simulink subsystem "Day1_Scenario_3_4"  (R2024a)
settings: Solver=VariableStepAuto  StartTime=0.0  StopTime=10.0  RelTol=1e-3
libraries: CarMaker4SL x3
settings Model: Creator=junhyung.cha  LastModifiedBy=User

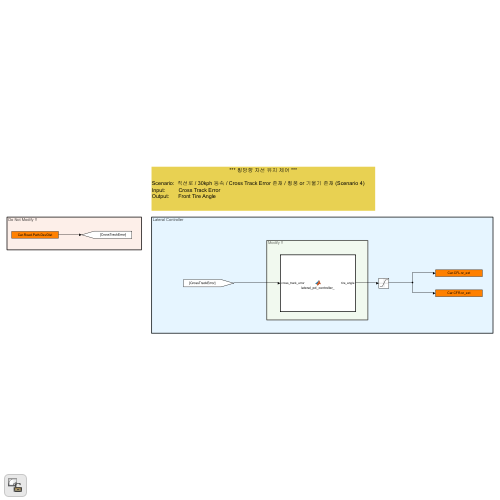
[thumbnail: Simulink's stored preview of the top-level diagram]
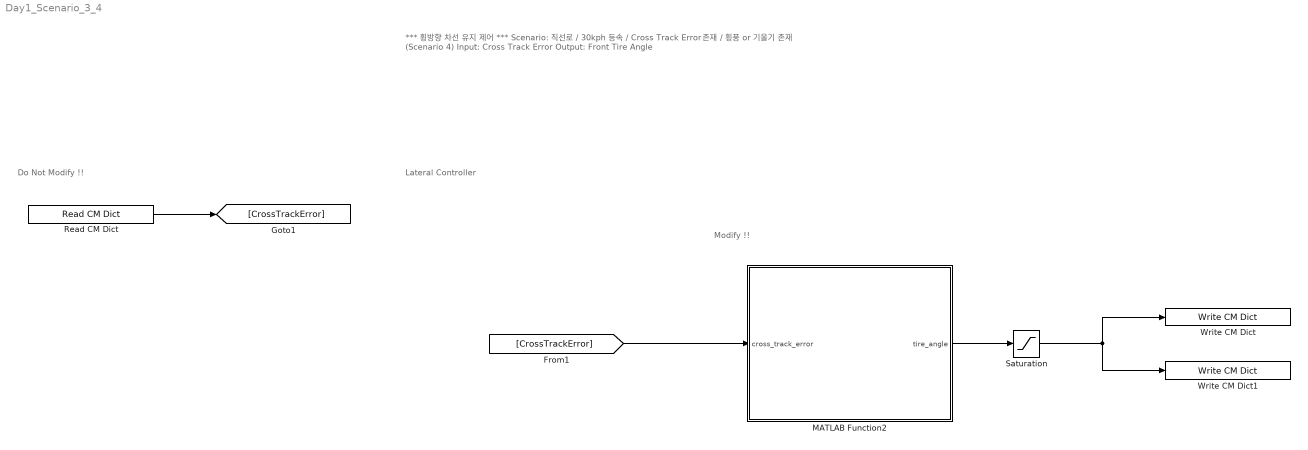
== system Day1_Scenario_3_4 ==
  note: Do Not Modify !!
  note: Modify !!
  note: Lateral Controller
  note: *** 횡방향 차선 유지 제어 ***
      |
      | Scenario: 직선로 / 30kph 등속 / Cross Track Error 존재 / 횡풍 or 기울기 존재 (Scenario 4)
      | Input: Cross Track Error
      | Output: Front Tire Angle
  MATLAB Function2 : MATLAB Function  TreatAsAtomicUnit=on
  Read CM Dict : CarMaker4SL/Read CM Dict  xname=Car.Road.Path.DevDist  xsync=off  xstime=Inherited
  Saturation : Saturate  UpperLimit=2  LowerLimit=-2
  Write CM Dict : CarMaker4SL/Write CM Dict  xname=Car.CFL.rz_ext  xsync=off
  Write CM Dict1 : CarMaker4SL/Write CM Dict  xname=Car.CFR.rz_ext  xsync=off
  wires:
  Read CM Dict/1 -> [CrossTrackError]
  MATLAB Function2/1(tire_angle) -> Saturation/1
  [CrossTrackError] -> MATLAB Function2/1(cross_track_error)
  Saturation/1 -> Write CM Dict/1, Write CM Dict1/1

== matlab function Day1_Scenario_3_4/MATLAB Function2 ==
  settings: updateMethod=DISCRETE  sampleTime=0.05
  data: cross_track_error input; tire_angle output
% PD 제어 코드

function tire_angle = lateral_pd_controller_(cross_track_error)

% Lateral PD Controller
% Input  : cross_track_error [m]
% Output : tire_angle [rad]

Ts = 0.01;     % sample time [s]

Kp = 0.03;     % P gain
Kd = 0.04;     % D gain

persistent prev_error

if isempty(prev_error)
    prev_error = cross_track_error;
end

% 현재 오차
error = cross_track_error;

% 오차 변화율
error_dot = (error - prev_error) / Ts;

% PD 제어
tire_angle = -(Kp * error + Kd * error_dot);

% 이전 오차 저장
prev_error = error;

end
